simulink model "AreaCoverageTestHarness"  (R2016a)
settings: Solver=FixedStepDiscrete  StartTime=0.0  StopTime=16  FixedStep=0.005  RelTol=1e-3
values from neighbouring files (symbols this model uses):
  EAST = 0    [AreaCoverageCalib.m]
  ERRVAL = 5    [AreaCoverageCalib.m]
  INIT_COMP_VALUE = SOUTH    (= 90)    [AreaCoverageCalib.m]
  INIT_X = round(roomSize/2)    [AreaCoverageCalib.m]
  INIT_Y = round(roomSize/2)    [AreaCoverageCalib.m]
  MAX_SPEED = 850    [AreaCoverageCalib.m]
  NORTH = 270    [AreaCoverageCalib.m]
  ROB_LENG = 30    [AreaCoverageCalib.m]
  ROB_WHEEL_R = .05    (= 0.05)    [AreaCoverageCalib.m]
  room = uint8(ones(roomSize , roomSize)*255)    [roomDrawing.m]
  roomSize = round(standardRoom_CM/ROBO_LENG + 2)    [roomDrawing.m]
  SAMPLE_TIME = 0.001    [AreaCoverageCalib.m]
  SOUTH = 90    [AreaCoverageCalib.m]
  STEP_SIZE = 5    [AreaCoverageCalib.m]
  WEST = 180    [AreaCoverageCalib.m]
undefined symbols (not defined in the file or in its folder): sigbuilder_block
(part 2 of 2)

== stateflow chart AreaCoverageTestHarness/Robot/EncoderTicksGenerator/SquareWaveCreatorLeft ==
  state BulbOn
    state Off
      entry:
      counter = 0;
      encoderTicks_BOOL = false;
      du:
      counter++;
    state On
      entry:
      counter = 0;
      encoderTicks_BOOL = true;
      du:
      counter++;
    (default) -> Off
    On -> Off : [counter >= 100]/counter = 0;
    Off -> On : [counter >= 100]/counter = 0;
  state BulbOff
    entry:
    encoderTicks_BOOL = 0;
  (default) -> BulbOff
  BulbOff -> BulbOn : [ControlSignal_BOOL_in]
  BulbOn -> BulbOff : [!ControlSignal_BOOL_in]
  data: ControlSignal_BOOL_in input; encoderTicks_BOOL output boolean; counter local uint16
